simulink model "ZAD1_1_Model"  (R2018a)
settings: Solver=ode45  StartTime=0.0  StopTime=tend  MaxStep=Tp  RelTol=1e-3
values from neighbouring files (symbols this model uses):
  initConditionsVel = [0; 0]    [ZAD0_SRManCw3_Init.m]
  invR = inv(R)    [ZAD0_SRManCw3_Init.m]
  Km = diag([km1; km2])    [ZAD0_SRManCw3_Init.m]
  U = [24.0; 24.0]    [ZAD0_SRManCw3_Init.m]
undefined symbols (not defined in the file or in its folder): initConditionsAcc, invEta
settings Model: Creator=szymon  LastModifiedBy=szymon

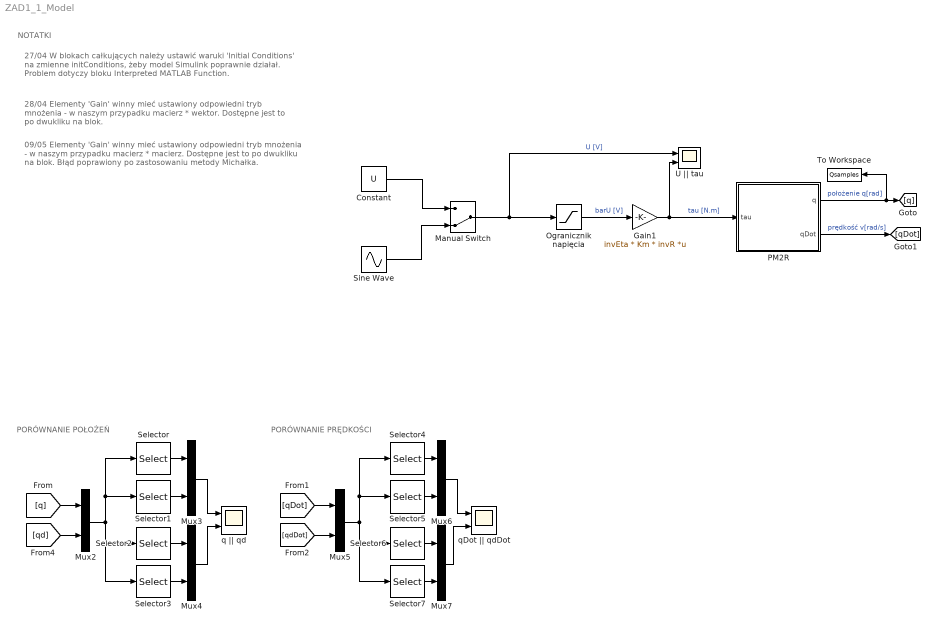
== system ZAD1_1_Model ==
  note: PORÓWNANIE POŁOŻEŃ
  note: NOTATKI
  note: 27/04 W blokach całkujących należy ustawić waruki
      | 'Initial Conditions' na zmienne initConditions, żeby model
      | Simulink poprawnie działał. Problem dotyczy bloku
      | Interpreted MATLAB Function.
  note: 28/04 Elementy 'Gain' winny mieć ustawiony odpowiedni tryb
      | mnożenia - w naszym przypadku macierz * wektor.
      | Dostępne jest to po dwukliku na blok.
  note: PORÓWNANIE PRĘDKOŚCI
  note: 09/05 Elementy 'Gain' winny mieć ustawiony odpowiedni tryb
      | mnożenia - w naszym przypadku macierz * macierz.
      | Dostępne jest to po dwukliku na blok. Błąd poprawiony po
      | zastosowaniu metody Michałka.
  Constant : Constant  Value=U
  Gain1 : Gain  Gain=invEta * Km * invR  Multiplication=Matrix(K*u)
  Manual Switch : ManualSwitch  CurrentSetting=0
  Mux{2..7} (6 alike) : Mux  Inputs=2
  Ogranicznik napięcia : Saturate  UpperLimit=24.0  LowerLimit=-24.0
  PM2R : Subsystem
  Selector : Selector  InputPortWidth=4  IndexOptions=Index vector (dialog)  Indices=[1]  OutputSizes=1
  Selector1 : Selector  InputPortWidth=4  IndexOptions=Index vector (dialog)  Indices=[3]  OutputSizes=1
  Selector2 : Selector  InputPortWidth=4  IndexOptions=Index vector (dialog)  Indices=[2]  OutputSizes=1
  Selector3 : Selector  InputPortWidth=4  IndexOptions=Index vector (dialog)  Indices=[4]  OutputSizes=1
  Selector4 : Selector  InputPortWidth=4  IndexOptions=Index vector (dialog)  Indices=[1]  OutputSizes=1
  Selector5 : Selector  InputPortWidth=4  IndexOptions=Index vector (dialog)  Indices=[3]  OutputSizes=1
  Selector6 : Selector  InputPortWidth=4  IndexOptions=Index vector (dialog)  Indices=[2]  OutputSizes=1
  Selector7 : Selector  InputPortWidth=4  IndexOptions=Index vector (dialog)  Indices=[4]  OutputSizes=1
  Sine Wave : Sin  Amplitude=U  SampleTime=0
  To Workspace : ToWorkspace  VariableName=Qsamples  SampleTime=-1
  U || tau : Scope  NumInputPorts=2
  q || qd : Scope  NumInputPorts=2
  qDot || qdDot : Scope  NumInputPorts=2
  wires:
  PM2R/2(qDot) -> [qDot]  "prędkość v[rad/s]"
  PM2R/1(q) -> [q], To Workspace/1  "położenie q[rad]"
  [q] -> Mux2/1
  [qd] -> Mux2/2
  Selector/1 -> Mux3/1
  Selector1/1 -> Mux3/2
  Selector2/1 -> Mux4/1
  Selector3/1 -> Mux4/2
  Mux2/1 -> Selector3/1, Selector2/1, Selector1/1, Selector/1
  Mux3/1 -> q || qd/1
  Mux4/1 -> q || qd/2
  Selector6/1 -> Mux7/1
  Mux6/1 -> qDot || qdDot/1
  Mux7/1 -> qDot || qdDot/2
  Selector7/1 -> Mux7/2
  [qDot] -> Mux5/1
  Selector5/1 -> Mux6/2
  [qdDot] -> Mux5/2
  Selector4/1 -> Mux6/1
  Mux5/1 -> Selector7/1, Selector6/1, Selector5/1, Selector4/1
  Gain1/1 -> U || tau/2, PM2R/1(tau)  "tau [N.m]"
  Manual Switch/1 -> U || tau/1, Ogranicznik napięcia/1  "U [V]"
  Constant/1 -> Manual Switch/1
  Sine Wave/1 -> Manual Switch/2
  Ogranicznik napięcia/1 -> Gain1/1  "barU [V]"

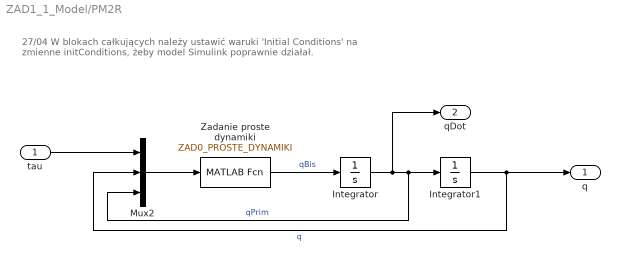
== system ZAD1_1_Model/PM2R ==
  note: 27/04 W blokach całkujących należy ustawić waruki 'Initial Conditions' na
      | zmienne initConditions, żeby model Simulink poprawnie działał.
  tau : Inport
  Integrator : Integrator  InitialCondition=initConditionsAcc
  Integrator1 : Integrator  InitialCondition=initConditionsVel
  Mux2 : Mux  Inputs=3
  Zadanie proste dynamiki : MATLABFcn  MATLABFcn=ZAD0_PROSTE_DYNAMIKI
  q : Outport
  qDot : Outport  Port=2
  wires:
  Zadanie proste dynamiki/1 -> Integrator/1  "qBis"
  Integrator/1 -> qDot/1, Mux2/3, Integrator1/1  "qPrim"
  Integrator1/1 -> q/1, Mux2/2  "q"
  tau/1 -> Mux2/1
  Mux2/1 -> Zadanie proste dynamiki/1
